simulink model "quadcopter_bes_kontrolera3d"  (R2015a)
settings: Solver=ode113  StartTime=0.0  StopTime=1500  RelTol=1e-3
libraries: simulink x5
settings Model: Creator=BLAGI  LastModifiedBy=BLAGI

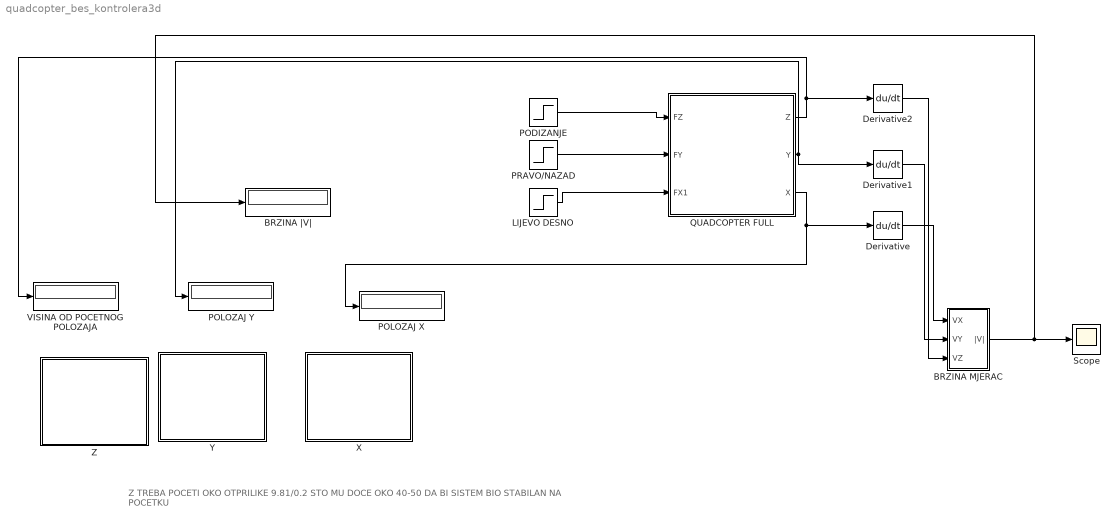
== system quadcopter_bes_kontrolera3d ==
  note: Z TREBA POCETI OKO OTPRILIKE 9.81/0.2 STO MU DOCE OKO 40-50 DA BI SISTEM BIO STABILAN NA POCETKU
  "\tLIJEVO DESNO" : Step  After=100  SampleTime=0
  "  POLOZAJ X" : Display
  "  POLOZAJ Y" : Display
  BRZINA MJERAC : Subsystem
  BRZINA |V| : Display
  Derivative : Derivative
  Derivative1 : Derivative
  Derivative2 : Derivative
  PODIZANJE : Step  After=87.7462  SampleTime=0
  PRAVO/NAZAD : Step  After=86.1721  SampleTime=0
  QUADCOPTER FULL : Subsystem
  Scope : Scope
      settings: TimeRange=1.74683918676622  YMin=0  YMax=34.08375  SaveName=ScopeData5
  VISINA OD POCETNOG POLOZAJA : Display
  X : Subsystem  DialogController=hmiCreateDDGDialog  IsWebBlock=on  mask(MathWorksWebBlock){webBlockId=fab8a9fa-ed1a-48d9-95db-399e88e1ca8e, webBlockType=continuousknob, ShowInLibBrowser=on, ShowInitialText=on, HMISrcModelName=quadcopter_bes_kontrolera3d}
      mask prompts: webBlockId "WebBlock Id"; webBlockType "WebBlock Type"; HMISrcModelName "Source Model"
      mask Help: helpview([docroot '/mapfiles/simulink.map'], 'hmi_knob')
      mask Display:
      | if strcmp(get_param(bdroot(gcb),'BlockDiagramType'), 'library')
      |     image([(matlabroot) '/toolbox/simulink/hmi/icons/ContinuousKnob.png']);
      | end
  Y : Subsystem  DialogController=hmiCreateDDGDialog  IsWebBlock=on  mask(MathWorksWebBlock){webBlockId=794acf75-0f82-4902-9a26-fb9d008e00b0, webBlockType=continuousknob, ShowInLibBrowser=on, ShowInitialText=on, HMISrcModelName=quadcopter_bes_kontrolera3d}
      mask prompts: webBlockId "WebBlock Id"; webBlockType "WebBlock Type"; HMISrcModelName "Source Model"
      mask Help: helpview([docroot '/mapfiles/simulink.map'], 'hmi_knob')
      mask Display:
      | if strcmp(get_param(bdroot(gcb),'BlockDiagramType'), 'library')
      |     image([(matlabroot) '/toolbox/simulink/hmi/icons/ContinuousKnob.png']);
      | end
  Z : Subsystem  DialogController=hmiCreateDDGDialog  IsWebBlock=on  mask(MathWorksWebBlock){webBlockId=14bd038a-bfe1-45b3-80ce-fd20c3c06831, webBlockType=continuousknob, ShowInLibBrowser=on, ShowInitialText=on, HMISrcModelName=quadcopter_bes_kontrolera3d}
      mask prompts: webBlockId "WebBlock Id"; webBlockType "WebBlock Type"; HMISrcModelName "Source Model"
      mask Help: helpview([docroot '/mapfiles/simulink.map'], 'hmi_knob')
      mask Display:
      | if strcmp(get_param(bdroot(gcb),'BlockDiagramType'), 'library')
      |     image([(matlabroot) '/toolbox/simulink/hmi/icons/ContinuousKnob.png']);
      | end
  wires:
  QUADCOPTER FULL/1(Z) -> Derivative2/1, VISINA OD POCETNOG POLOZAJA/1
  QUADCOPTER FULL/2(Y) -> Derivative1/1, "  POLOZAJ Y"/1
  QUADCOPTER FULL/3(X) -> "  POLOZAJ X"/1, Derivative/1
  Derivative2/1 -> BRZINA MJERAC/3(VZ)
  Derivative1/1 -> BRZINA MJERAC/2(VY)
  Derivative/1 -> BRZINA MJERAC/1(VX)
  BRZINA MJERAC/1(" |V|") -> BRZINA |V|/1, Scope/1
  PODIZANJE/1 -> QUADCOPTER FULL/1(FZ)
  PRAVO/NAZAD/1 -> QUADCOPTER FULL/2(FY)
  "\tLIJEVO DESNO"/1 -> QUADCOPTER FULL/3(FX1)

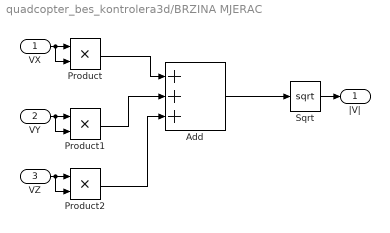
== system quadcopter_bes_kontrolera3d/BRZINA MJERAC ==
  VX : Inport
  VY : Inport  Port=2
  VZ : Inport  Port=3
  Add : Sum  Inputs=+++
  Product : Product
  Product1 : Product
  Product2 : Product
  Sqrt : Sqrt  SaturateOnIntegerOverflow=on
  " |V|" : Outport
  wires:
  Product1/1 -> Add/2
  Product/1 -> Add/1
  Add/1 -> Sqrt/1
  Product2/1 -> Add/3
  Sqrt/1 -> " |V|"/1
  VY/1 -> Product1/2, Product1/1
  VZ/1 -> Product2/2, Product2/1
  VX/1 -> Product/2, Product/1

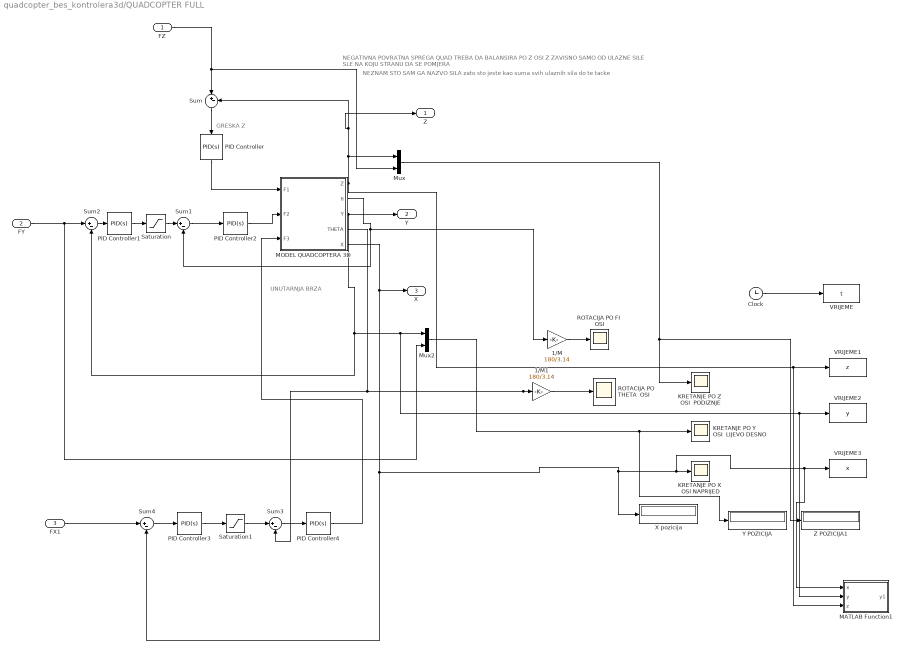
== system quadcopter_bes_kontrolera3d/QUADCOPTER FULL ==
  note: UNUTARNJA BRZA
  note: GRESKA Z
  note: NEZNAM STO SAM GA NAZVO SILA zato sto jeste kao suma svih ulaznih sila do te tacke
  note: NEGATIVNA POVRATNA SPREGA QUAD TREBA DA BALANSIRA PO Z OSI Z ZAVISNO SAMO OD ULAZNE SILE SLE NA KOJU STRANU DA SE POMJERA
  FZ : Inport
  FY : Inport  Port=2
  FX1 : Inport  Port=3
  1/M : Gain  Gain=180/3.14
  1/M1 : Gain  Gain=180/3.14
  Clock : Clock
  KRETANJE PO X  OSI NAPRIJED : Scope
      settings: YMin=49.9993  YMax=50.0008  SaveName=ScopeData4
  KRETANJE PO Y  OSI  LIJEVO DESNO : Scope
      settings: SaveName=ScopeData2
  KRETANJE PO Z  OSI  PODIZNJE : Scope
  MATLAB Function1 : MATLAB Function  TreatAsAtomicUnit=on
  "MODEL QUADCOPTERA 3D " : Subsystem
  Mux : Mux  Inputs=2
  Mux2 : Mux  Inputs=2
  PID Controller : simulink/Continuous/PID Controller  Controller=PID  TimeDomain=Continuous-time  SampleTime=-1  IntegratorMethod=Forward Euler  FilterMethod=Forward Euler  Form=Parallel  UseFilter=on  ControllerParametersSource=internal  P=0.0707609084607024  I=0.00457273854837388  D=0.268877039592949  N=7.52857471853222  InitialConditionSource=internal  InitialConditionForIntegrator=0  InitialConditionForFilter=0  ExternalReset=none  LimitOutput=off  UpperSaturationLimit=inf  LowerSaturationLimit=-inf  LinearizeAsGain=on  AntiWindupMode=none  Kb=1  TrackingMode=off  Kt=1  PParamMin=[]  PParamMax=[]  IParamMin=[]  IParamMax=[]  DParamMin=[]  DParamMax=[]  NParamMin=[]  NParamMax=[]  KbParamMin=[]  KbParamMax=[]  KtParamMin=[]  KtParamMax=[]  POutMin=[]  POutMax=[]  IOutMin=[]  IOutMax=[]  DOutMin=[]  DOutMax=[]  NOutMin=[]  NOutMax=[]  KbOutMin=[]  KbOutMax=[]  KtOutMin=[]  KtOutMax=[]  IntegratorOutMin=[]  IntegratorOutMax=[]  FilterOutMin=[]  FilterOutMax=[]  SumOutMin=[]  SumOutMax=[]  SumI1OutMin=[]  SumI1OutMax=[]  SumI2OutMin=[]  SumI2OutMax=[]  SumI3OutMin=[]  SumI3OutMax=[]  SumDOutMin=[]  SumDOutMax=[]  SaturationOutMin=[]  SaturationOutMax=[]  IntegratorContinuousStateAttributes=''  IntegratorStateMustResolveToSignalObject=off  IntegratorRTWStateStorageClass=Auto  FilterContinuousStateAttributes=''  FilterStateMustResolveToSignalObject=off  FilterRTWStateStorageClass=Auto  DifferentiatorICPrevScaledInput=0  DifferentiatorOutMin=[]  DifferentiatorOutMax=[]
  PID Controller1 : simulink/Continuous/PID Controller  Controller=PID  TimeDomain=Continuous-time  SampleTime=-1  IntegratorMethod=Forward Euler  FilterMethod=Forward Euler  Form=Parallel  UseFilter=on  ControllerParametersSource=internal  P=3  I=0  D=5  N=23.0374094575144  InitialConditionSource=internal  InitialConditionForIntegrator=0  InitialConditionForFilter=0  ExternalReset=none  LimitOutput=off  UpperSaturationLimit=inf  LowerSaturationLimit=-inf  LinearizeAsGain=on  AntiWindupMode=none  Kb=1  TrackingMode=off  Kt=1  PParamMin=[]  PParamMax=[]  IParamMin=[]  IParamMax=[]  DParamMin=[]  DParamMax=[]  NParamMin=[]  NParamMax=[]  KbParamMin=[]  KbParamMax=[]  KtParamMin=[]  KtParamMax=[]  POutMin=[]  POutMax=[]  IOutMin=[]  IOutMax=[]  DOutMin=[]  DOutMax=[]  NOutMin=[]  NOutMax=[]  KbOutMin=[]  KbOutMax=[]  KtOutMin=[]  KtOutMax=[]  IntegratorOutMin=[]  IntegratorOutMax=[]  FilterOutMin=[]  FilterOutMax=[]  SumOutMin=[]  SumOutMax=[]  SumI1OutMin=[]  SumI1OutMax=[]  SumI2OutMin=[]  SumI2OutMax=[]  SumI3OutMin=[]  SumI3OutMax=[]  SumDOutMin=[]  SumDOutMax=[]  SaturationOutMin=[]  SaturationOutMax=[]  IntegratorContinuousStateAttributes=''  IntegratorStateMustResolveToSignalObject=off  IntegratorRTWStateStorageClass=Auto  FilterContinuousStateAttributes=''  FilterStateMustResolveToSignalObject=off  FilterRTWStateStorageClass=Auto  DifferentiatorICPrevScaledInput=0  DifferentiatorOutMin=[]  DifferentiatorOutMax=[]
  PID Controller2 : simulink/Continuous/PID Controller  Controller=PID  TimeDomain=Continuous-time  SampleTime=-1  IntegratorMethod=Forward Euler  FilterMethod=Forward Euler  Form=Parallel  UseFilter=on  ControllerParametersSource=internal  P=150  I=0  D=50  N=41.2028568285721  InitialConditionSource=internal  InitialConditionForIntegrator=0  InitialConditionForFilter=0  ExternalReset=none  LimitOutput=off  UpperSaturationLimit=inf  LowerSaturationLimit=-inf  LinearizeAsGain=on  AntiWindupMode=none  Kb=1  TrackingMode=off  Kt=1  PParamMin=[]  PParamMax=[]  IParamMin=[]  IParamMax=[]  DParamMin=[]  DParamMax=[]  NParamMin=[]  NParamMax=[]  KbParamMin=[]  KbParamMax=[]  KtParamMin=[]  KtParamMax=[]  POutMin=[]  POutMax=[]  IOutMin=[]  IOutMax=[]  DOutMin=[]  DOutMax=[]  NOutMin=[]  NOutMax=[]  KbOutMin=[]  KbOutMax=[]  KtOutMin=[]  KtOutMax=[]  IntegratorOutMin=[]  IntegratorOutMax=[]  FilterOutMin=[]  FilterOutMax=[]  SumOutMin=[]  SumOutMax=[]  SumI1OutMin=[]  SumI1OutMax=[]  SumI2OutMin=[]  SumI2OutMax=[]  SumI3OutMin=[]  SumI3OutMax=[]  SumDOutMin=[]  SumDOutMax=[]  SaturationOutMin=[]  SaturationOutMax=[]  IntegratorContinuousStateAttributes=''  IntegratorStateMustResolveToSignalObject=off  IntegratorRTWStateStorageClass=Auto  FilterContinuousStateAttributes=''  FilterStateMustResolveToSignalObject=off  FilterRTWStateStorageClass=Auto  DifferentiatorICPrevScaledInput=0  DifferentiatorOutMin=[]  DifferentiatorOutMax=[]
  PID Controller3 : simulink/Continuous/PID Controller  Controller=PID  TimeDomain=Continuous-time  SampleTime=-1  IntegratorMethod=Forward Euler  FilterMethod=Forward Euler  Form=Parallel  UseFilter=on  ControllerParametersSource=internal  P=3  I=0  D=5  N=5.66031803135333  InitialConditionSource=internal  InitialConditionForIntegrator=0  InitialConditionForFilter=0  ExternalReset=none  LimitOutput=off  UpperSaturationLimit=inf  LowerSaturationLimit=-inf  LinearizeAsGain=on  AntiWindupMode=none  Kb=1  TrackingMode=off  Kt=1  PParamMin=[]  PParamMax=[]  IParamMin=[]  IParamMax=[]  DParamMin=[]  DParamMax=[]  NParamMin=[]  NParamMax=[]  KbParamMin=[]  KbParamMax=[]  KtParamMin=[]  KtParamMax=[]  POutMin=[]  POutMax=[]  IOutMin=[]  IOutMax=[]  DOutMin=[]  DOutMax=[]  NOutMin=[]  NOutMax=[]  KbOutMin=[]  KbOutMax=[]  KtOutMin=[]  KtOutMax=[]  IntegratorOutMin=[]  IntegratorOutMax=[]  FilterOutMin=[]  FilterOutMax=[]  SumOutMin=[]  SumOutMax=[]  SumI1OutMin=[]  SumI1OutMax=[]  SumI2OutMin=[]  SumI2OutMax=[]  SumI3OutMin=[]  SumI3OutMax=[]  SumDOutMin=[]  SumDOutMax=[]  SaturationOutMin=[]  SaturationOutMax=[]  IntegratorContinuousStateAttributes=''  IntegratorStateMustResolveToSignalObject=off  IntegratorRTWStateStorageClass=Auto  FilterContinuousStateAttributes=''  FilterStateMustResolveToSignalObject=off  FilterRTWStateStorageClass=Auto  DifferentiatorICPrevScaledInput=0  DifferentiatorOutMin=[]  DifferentiatorOutMax=[]
  PID Controller4 : simulink/Continuous/PID Controller  Controller=PID  TimeDomain=Continuous-time  SampleTime=-1  IntegratorMethod=Forward Euler  FilterMethod=Forward Euler  Form=Parallel  UseFilter=on  ControllerParametersSource=internal  P=150  I=0  D=50  N=41.2028568285721  InitialConditionSource=internal  InitialConditionForIntegrator=0  InitialConditionForFilter=0  ExternalReset=none  LimitOutput=off  UpperSaturationLimit=inf  LowerSaturationLimit=-inf  LinearizeAsGain=on  AntiWindupMode=none  Kb=1  TrackingMode=off  Kt=1  PParamMin=[]  PParamMax=[]  IParamMin=[]  IParamMax=[]  DParamMin=[]  DParamMax=[]  NParamMin=[]  NParamMax=[]  KbParamMin=[]  KbParamMax=[]  KtParamMin=[]  KtParamMax=[]  POutMin=[]  POutMax=[]  IOutMin=[]  IOutMax=[]  DOutMin=[]  DOutMax=[]  NOutMin=[]  NOutMax=[]  KbOutMin=[]  KbOutMax=[]  KtOutMin=[]  KtOutMax=[]  IntegratorOutMin=[]  IntegratorOutMax=[]  FilterOutMin=[]  FilterOutMax=[]  SumOutMin=[]  SumOutMax=[]  SumI1OutMin=[]  SumI1OutMax=[]  SumI2OutMin=[]  SumI2OutMax=[]  SumI3OutMin=[]  SumI3OutMax=[]  SumDOutMin=[]  SumDOutMax=[]  SaturationOutMin=[]  SaturationOutMax=[]  IntegratorContinuousStateAttributes=''  IntegratorStateMustResolveToSignalObject=off  IntegratorRTWStateStorageClass=Auto  FilterContinuousStateAttributes=''  FilterStateMustResolveToSignalObject=off  FilterRTWStateStorageClass=Auto  DifferentiatorICPrevScaledInput=0  DifferentiatorOutMin=[]  DifferentiatorOutMax=[]
  ROTACIJA PO FI  OSI : Scope
      settings: TimeRange=0.009047248944913378  YMin=-4.230680640277781  YMax=-4.194058720833336
  ROTACIJA PO THETA  OSI : Scope
      settings: TimeRange=45.82848796997469  YMin=0.793  YMax=0.806  SaveName=ScopeData3
  Saturation : Saturate
  Saturation1 : Saturate
  Sum{,1..4} (5 alike) : Sum  Inputs=|+-
  VRIJEME : ToWorkspace  VariableName=t  SaveFormat=Timeseries  SampleTime=-1
  VRIJEME1 : ToWorkspace  VariableName=z  SaveFormat=Timeseries  SampleTime=-1
  VRIJEME2 : ToWorkspace  VariableName=y  SaveFormat=Timeseries  SampleTime=-1
  VRIJEME3 : ToWorkspace  VariableName=x  SaveFormat=Timeseries  SampleTime=-1
  X pozicija : Display
  Y POZICIJA : Display
  Z POZICIJA1 : Display
  Z : Outport
  Y : Outport  Port=2
  X : Outport  Port=3
  wires:
  PID Controller4/1 -> "MODEL QUADCOPTERA 3D "/3(F3)
  Sum3/1 -> PID Controller4/1
  Sum4/1 -> PID Controller3/1
  FX1/1 -> Sum4/1
  PID Controller1/1 -> Saturation/1
  Mux2/1 -> KRETANJE PO Y  OSI  LIJEVO DESNO/1, Y POZICIJA/1
  "MODEL QUADCOPTERA 3D "/2(fi) -> Sum1/2, 1/M/1
  PID Controller/1 -> "MODEL QUADCOPTERA 3D "/1(F1)
  PID Controller2/1 -> "MODEL QUADCOPTERA 3D "/2(F2)
  Saturation/1 -> Sum1/1
  Sum1/1 -> PID Controller2/1
  FY/1 -> Mux2/2, Sum2/1
  "MODEL QUADCOPTERA 3D "/3(Y) -> MATLAB Function1/2(y), VRIJEME2/1, Mux2/1, Sum2/2, Y/1
  FZ/1 -> Mux/2, Sum/1
  Sum2/1 -> PID Controller1/1
  Sum/1 -> PID Controller/1
  Clock/1 -> VRIJEME/1
  Mux/1 -> KRETANJE PO Z  OSI  PODIZNJE/1, Z POZICIJA1/1
  "MODEL QUADCOPTERA 3D "/1(Z) -> MATLAB Function1/3(z), VRIJEME1/1, Mux/1, Z/1, Sum/2
  "MODEL QUADCOPTERA 3D "/4(THETA) -> 1/M1/1, Sum3/2
  PID Controller3/1 -> Saturation1/1
  Saturation1/1 -> Sum3/1
  1/M/1 -> ROTACIJA PO FI  OSI/1
  1/M1/1 -> ROTACIJA PO THETA  OSI/1
  "MODEL QUADCOPTERA 3D "/5(X) -> X/1, X pozicija/1, MATLAB Function1/1(x), VRIJEME3/1, KRETANJE PO X  OSI NAPRIJED/1, Sum4/2

== system quadcopter_bes_kontrolera3d/X ==

== system quadcopter_bes_kontrolera3d/Y ==

== system quadcopter_bes_kontrolera3d/Z ==

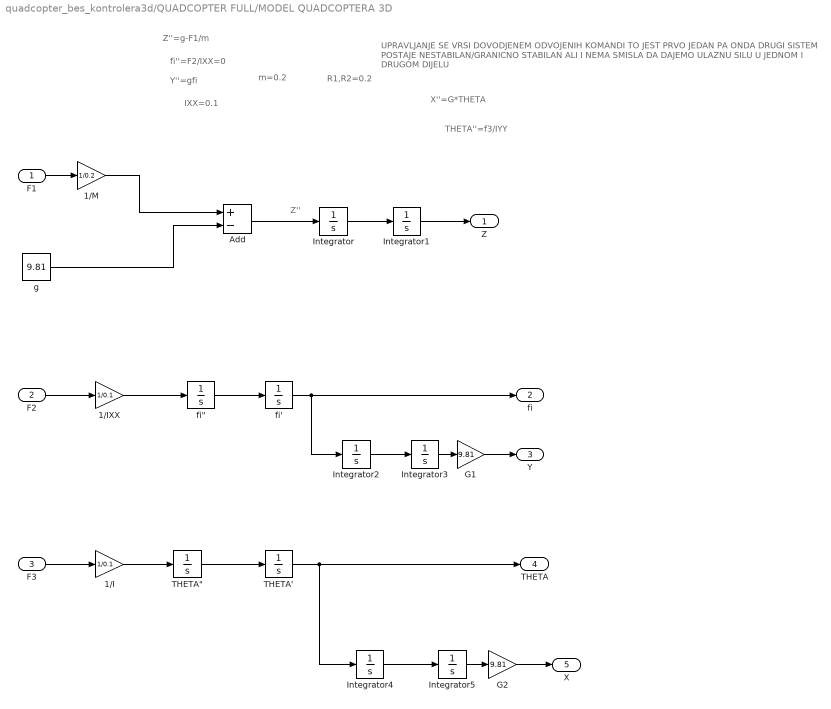
== system quadcopter_bes_kontrolera3d/QUADCOPTER FULL/MODEL QUADCOPTERA 3D  ==
  note: UPRAVLJANJE SE VRSI DOVODJENEM ODVOJENIH KOMANDI TO JEST PRVO JEDAN PA ONDA DRUGI
      | SISTEM POSTAJE NESTABILAN/GRANICNO STABILAN ALI I NEMA SMISLA DA DAJEMO ULAZNU SILU U JEDNOM I DRUGOM DIJELU
  note: THETA''=f3/IYY
  note: X''=G*THETA
  note: R1,R2=0.2
  note: m=0.2
  note: IXX=0.1
  note: Z''
  note: Y''=gfi
  note: fi''=F2/IXX=0
  note: Z''=g-F1/m
  F1 : Inport
  F2 : Inport  Port=2
  F3 : Inport  Port=3
  1/I : Gain  Gain=1/0.1
  1/IXX : Gain  Gain=1/0.1
  1/M : Gain  Gain=1/0.2
  Add : Sum  Inputs=+-
  G1 : Gain  Gain=9.81
  G2 : Gain  Gain=9.81
  Integrator : Integrator  UpperSaturationLimit=1  LowerSaturationLimit=-1  IgnoreLimit=on
  Integrator1 : Integrator
  Integrator2 : Integrator  LimitOutput=on  UpperSaturationLimit=1  LowerSaturationLimit=-1
  Integrator3 : Integrator
  Integrator4 : Integrator  LimitOutput=on  UpperSaturationLimit=1  LowerSaturationLimit=-1
  Integrator5 : Integrator
  "THETA\"" : Integrator
  THETA' : Integrator
  "fi\"" : Integrator
  fi' : Integrator
  g : Constant  Value=9.81
  Z : Outport
  fi : Outport  Port=2
  Y : Outport  Port=3
  THETA : Outport  Port=4
  X : Outport  Port=5
  wires:
  G1/1 -> Y/1
  Integrator2/1 -> Integrator3/1
  F1/1 -> 1/M/1
  1/IXX/1 -> "fi\""/1
  Integrator/1 -> Integrator1/1
  Add/1 -> Integrator/1
  g/1 -> Add/2
  Integrator3/1 -> G1/1
  "fi\""/1 -> fi'/1
  fi'/1 -> fi/1, Integrator2/1
  Integrator1/1 -> Z/1
  1/M/1 -> Add/1
  F2/1 -> 1/IXX/1
  1/I/1 -> "THETA\""/1
  F3/1 -> 1/I/1
  "THETA\""/1 -> THETA'/1
  THETA'/1 -> Integrator4/1, THETA/1
  Integrator4/1 -> Integrator5/1
  Integrator5/1 -> G2/1
  G2/1 -> X/1

== matlab function quadcopter_bes_kontrolera3d/QUADCOPTER FULL/MATLAB Function1 ==
  data: x input; y input; z input; y1 output
function y1 = fcn(x,y,z)
%#codegen
plot3(x,y,z,'O');
hold on
y1 =  1;
